simulink model "vandevusse"  (R2020b)
settings: Solver=VariableStepAuto  StartTime=0.0  StopTime=0.5  MaxStep=1e-3  MinStep=1e-4  RelTol=1e-3
settings Model: Creator=Gustavo Caldas  LastModifiedBy=Gustavo Caldas

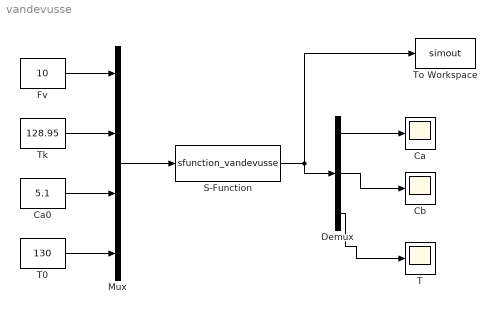
== system vandevusse ==
  Ca : Scope
  Ca0 : Constant  Value=5.1
  Cb : Scope
  Demux : Demux  Outputs=3
  Fv : Constant  Value=10
  Mux : Mux
  S-Function : S-Function  FunctionName=sfunction_vandevusse  SFunctionDeploymentMode=off  EnableBusSupport=off
  T : Scope
  T0 : Constant  Value=130
  Tk : Constant  Value=128.95
  To Workspace : ToWorkspace  VariableName=simout  SaveFormat=Timeseries  SampleTime=-1
  wires:
  Ca0/1 -> Mux/3
  Mux/1 -> S-Function/1
  Tk/1 -> Mux/2
  S-Function/1 -> To Workspace/1, Demux/1
  Demux/2 -> Cb/1
  T0/1 -> Mux/4
  Demux/1 -> Ca/1
  Fv/1 -> Mux/1
  Demux/3 -> T/1
